simulink model "HIL_Testing_SW_amantest"  (Simulink 7.5)
settings: Solver=ode1  StartTime=0.0  StopTime=Inf  FixedStep=0.001  RelTol=1e-3
PostLoadFcn:
  | , if any(exist('dsrtsu_mdlpostloadfcn', 'file') == [2, 3, 6]), try dsrtsu_mdlpostloadfcn('Execute', bdroot); catch fprintf('Error in PostLoadFcn (dsrtsu_mdlpostloadfcn) for model "%s":\n %s\n', bdroot, lasterr); end, end,
undefined symbols (not defined in the file): CeBSER_Cnt_NumTempAxisPts, ChargeCord, ChargeCord_Control, ChargeToSOCCurr, ChrgCurrLim, CrntSens1Fine, CS_SOCSetPt, CyclerMaxChrgPwr, CyclerMaxDschrgPwr, deltaAhr, Drive_1, Drive_10, Drive_11, Drive_12, Drive_13, Drive_14, Drive_15, Drive_16, Drive_17, Drive_18, Drive_19, Drive_2, Drive_20, Drive_21, Drive_22, Drive_23, Drive_24, Drive_25, Drive_26, Drive_27, Drive_28, Drive_29, Drive_3, Drive_30, Drive_31, Drive_32, Drive_33, Drive_34, Drive_35, Drive_36, Drive_37, Drive_38, Drive_39, Drive_4, Drive_40, Drive_41, Drive_42, Drive_43, Drive_44, Drive_45, Drive_46, Drive_47, Drive_48, Drive_49, Drive_5, Drive_50, Drive_51, Drive_6, Drive_7, Drive_8 ... (+50)
libraries: simulink x129, rtican x50, rti2211sailib x5, rti2211serlib x5, rti2202miolib x3
(part 8 of 23)

== system HIL_Testing_SW_amantest/RX/Read BAS3/Read PTEX ==
  PPEI_High_Vlt_Battery_Vlt_Status1 : rtican/RTICAN Receive (RX)   SystemSampleTime=-1  Reserved1=[]  Reserved2=[]  Reserved3=[]  Reserved4=[]  SfcnMessage=[]  Msg_Struct=[]  BoardTypeNo=[]  BoardNo=[]  ChannelNo=[]  Parameters=[]  DialogFcn=[]  UnitName=[]  Revision=[]  UnitValues=[]  DSProperties=struct('RTI',struct('Version',uint32(5),'BlockType',struct('isSLSource',uint8(1),'isSLSink',uint8(1),'isHWSource',uint8(0),'isHWSink',uint8(0),'isSetup',uint8(0),'isInline',uint8(1),'isNonInline',uint8(0),'isInterrupt',uint8(0),'isChannelwise',uint8(0)),'IOBoardType','RTICAN','UnitType','MESSAGE','Identifier','RX','DialogType','MSVC','BlockSet','RTICAN','SlaveProcessor','CAN'))  RTIBlockInterface=struct('OutputPortsWidth',int32([1 1 1 1 1 1 1 1]),'OutputPortsActive',[1 1 1 1 1 1 1 1],'OutputPortsName',{{'HVBatVltLwLmtCrnk','HVBatVltLwLmtCrnkV','HVBatVltLwLmt','HVBatVltLwLmtV','HVBatVltUpLmt','HVBatVltUpLmtV','HVBatPackPrcdVltg','HVBatPackPrcdVltgV'}},'OutputPortsDataType',{{'SS_DOUBLE','SS_DOUBLE','SS_DOUBLE','SS_DOUBLE','SS_DOUBLE','SS_DOUBLE','SS_DOUBLE','SS_DOUBLE'}},'OutputPortsLabel',{{'HVBatVltLwLmtCrnk','HVBatVltLwLmtCrnkV','HVBatVltLwLmt','HVBatVltLwLmtV','HVBatVltUpLmt','HVBatVltUpLmtV','HVBatPackPrcdVltg','HVBatPackPrcdVltgV'}},'OutputPortsLabelMode','ON','InputPortsWidth',int32(0),'InputPortsActive',0,'DialogFcn','rtican_message_interface_gui','BlockDisplay',{{'','center'}},'IconTransparency','on','ParameterTunableNames',{{}},'InitLevel',3,'BlockName',struct('Token',{{'PPEI_High_Vlt_Battery_Vlt_Status'}}),'SampleTime',{{-1}},'TriggerPort',{{'none'}},'EnablePort',{{'none'}})  RTIBlockParameters=struct('BoardTypeNo',{{4302,'OFF',[]}},'BoardNo',{{1,'ON',[1 16]}},'ChannelNo',{{2,'ON',[1 4]}},'Parameters',{{struct('DataFileSupport',struct('DataFileSelectedMaster',1,'DataFileSelectedLocal',1,'DataFileName',['c:\data\databases\6.4.1\globala - pe.dbc|'],'DataFileDate',['24-Apr-2014 15:33:48'],'SelectedFile',['..\databases\8.4.5 (140425)\globala - pe.dbc'],'InterfaceFcn','rtican_dbc_file_parser'),'Options',struct('StatusSelected',0,'TimeSelected',0,'DeltaTimeSelected',0,'BytePortSelected',0,'MessageLengthSelected',0,'TriggerPort',struct('Selected',0,'TriggerType',0),'UserCoding',struct('Selected',0,'InterfaceFile','UserDecodingFile','FcnName','UserDecodeFcn','InportSelected',0,'InportWidth',1,'OutportSelected',0,'OutportWidth',1),'EnablePortSelected',0,'SignalOnPortnameSelected',1,'UseRXService',0),'Message',struct('MsgOnBlocknameSelected',1,'MsgName','PPEI_High_Vlt_Battery_Vlt_Status','MsgIdFormat',0,'MsgId',983,'MsgLength',8,'NumSignals',8,'SampleTime',-1,'Signal',struct('SgnName',{'HVBatVltLwLmtCrnk','HVBatVltLwLmtCrnkV','HVBatVltLwLmt','HVBatVltLwLmtV','HVBatVltUpLmt','HVBatVltUpLmtV','HVBatPackPrcdVltg','HVBatPackPrcdVltgV'},'SgnStartBit',{0,10,16,26,32,42,48,58},'SgnLength',{10,1,10,1,10,1,10,1},'ByteLayout',{2,2,2,2,2,2,2,2},'Factor',{0.52,1,0.52,1,0.52,1,0.52,1},'Offset',{0,0,0,0,0,0,0,0},'SgnComment',{'','','','','','','',''},'SgnUnit',{'V','','V','','V','','V',''},'Min',{0,0,0,0,0,0,0,0},'Max',{531.96,1,531.96,1,531.96,1,531.96,1},'SgnType',{0,0,0,0,0,0,0,0},'SLDataType',{'SS_DOUBLE','SS_DOUBLE','SS_DOUBLE','SS_DOUBLE','SS_DOUBLE','SS_DOUBLE','SS_DOUBLE','SS_DOUBLE'},'DataType',{0,0,0,0,0,0,0,0},'ModeValue',{-1,-1,-1,-1,-1,-1,-1,-1}),'MsgIdNumFormat',0,'MsgComment',{{''}}),'Version',1.2,'general',struct('isFromLib',0)),'OFF',[]}},'GroupId',{{struct('Group',{{'RTICAN'}},'No',5,'Behavior',{{'NAMECHANGE'}},'BlockType',{{'SINK'}},'NameChangeFlag',0),'OFF',[]}},'SFcnRTICANMessage',{{struct('MsgType','RX','SFcnPortType','Scalar','MsgName','PPEI_High_Vlt_Battery_Vlt_Status','MsgIdFormat','STD','MsgId',983,'MsgLength',8,'NumSignals',8,'SampleTime',-1,'Signal',struct('SgnName',{'HVBatVltLwLmtCrnk','HVBatVltLwLmtCrnkV','HVBatVltLwLmt','HVBatVltLwLmtV','HVBatVltUpLmt','HVBatVltUpLmtV','HVBatPackPrcdVltg','HVBatPackPrcdVltgV'},'SgnStartBit',{0,10,16,26,32,42,48,58},'SgnLength',{10,1,10,1,10,1,10,1},'ByteLayout',{['motorola back.'],['motorola back.'],['motorola back.'],['motorola back.'],['motorola back.'],['motorola back.'],['motorola back.'],['motorola back.']},'Factor',{0.52,1,0.52,1,0.52,1,0.52,1},'Offset',{0,0,0,0,0,0,0,0},'SgnType',{'standard','standard','standard','standard','standard','standard','standard','standard'},'SLDataType',{'SS_DOUBLE','SS_DOUBLE','SS_DOUBLE','SS_DOUBLE','SS_DOUBLE','SS_DOUBLE','SS_DOUBLE','SS_DOUBLE'},'DataType',{['unsigned int'],['unsigned int'],['unsigned int'],['unsigned int'],['unsigned int'],['unsigned int'],['unsigned int'],['unsigned int']},'ModeValue',{-1,-1,-1,-1,-1,-1,-1,-1}),'StatusSelected','no','TimeSelected','no','DeltaTimeSelected','no','BytePortSelected','no','MessageLengthSelected','no','TriggerPort',struct('Selected','no','TriggerType',0),'UserCoding',struct('Selected','no','InterfaceFile','UserDecodingFile','FcnName','UserDecodeFcn','InportSelected','no','InportWidth',1,'OutportSelected','no','OutportWidth',1),'EnablePortSelected','no','UseRXService','no','BoardType','DS4302','BoardNo',1,'ControllerNo',2),'OFF',[]}},'TLCFileName',{{'rtican_rx_message','OFF',[]}})  RTISFcnParameters=struct('SFcnRTICANMessage','struct','TLCFileName','char')  RTIBlockParaDefault=struct('BoardTypeNo',4302,'BoardNo',1,'ChannelNo',1,'Parameters',struct('DataFileSupport',struct('DataFileSelectedMaster',0,'DataFileSelectedLocal',0,'DataFileName','','DataFileDate','','SelectedFile',['<no file selected>']),'Options',struct('StatusSelected',1,'TimeSelected',1,'DeltaTimeSelected',1,'BytePortSelected',0,'MessageLengthSelected',0,'TriggerPort',struct('Selected',0,'TriggerType','rising'),'UserCoding',struct('Selected',0,'InterfaceFile','UserDecodingFile','FcnName','UserDecodeFcn','InportSelected',0,'InportWidth',1,'OutportSelected',0,'OutportWidth',1),'EnablePortSelected',0,'SignalOnPortnameSelected',1,'UseRXService',0),'Message',struct('MsgOnBlocknameSelected',0,'MsgName',['RX Message'],'MsgIdFormat',0,'MsgId',100,'MsgLength',8,'NumSignals',1,'SampleTime',-1,'Signal',struct('SgnName',['RX signal'],'SgnStartBit',0,'SgnLength',8,'SgnType',0,'ModeValue',-1,'DataType',0,'SLDataType','SS_DOUBLE','ByteLayout',0,'Factor',1,'Offset',0,'Min',0,'Max',255,'SgnComment',{{}},'SgnUnit',''),'MsgIdNumFormat',0,'MsgComment',{{''}}),'Version',1.2,'general',struct('isFromLib',1)),'GroupId',struct('Group',{{'RTICAN'}},'No',1,'Behavior',{{'NAMECHANGE'}},'BlockType',{{'SINK'}},'NameChangeFlag',0),'SFcnRTICANMessage',struct('MsgType','RX','MsgName',['RX Message'],'MsgIdFormat','STD','MsgId',100,'MsgLength',8,'NumSignals',1,'SampleTime',-1,'Signal',struct('SgnName',['RX signal'],'SgnStartBit',0,'SgnLength',8,'SgnType','standard','ModeValue',-1,'DataType',['unsigned int'],'ByteLayout',['little endian'],'SLDataType','SS_DOUBLE','Factor',1,'Offset',0),'StatusSelected','yes','TimeSelected','yes','DeltaTimeSelected','yes','BytePortSelected','no','MessageLengthSelected','no','EnablePortSelected','no','UserCoding',struct('Selected','no','InterfaceFile','UserDecodingFile','FcnName','UserDecodeFcn','InportSelected','no','InportWidth',1,'OutportSelected','no','OutportWidth',1),'TriggerPort',struct('Selected','no','TriggerType','rising'),'UseRXService','no','BoardType','DS4302','BoardNo',1,'ControllerNo',1,'SFcnPortType','Scalar'),'TLCFileName','rtican_rx_message')
      settings: AttributesFormatString=Group Id: RTICAN5\n
  PPEI_High_Volt_Batt_Current_Stat1 : rtican/RTICAN Receive (RX)   SystemSampleTime=-1  Reserved1=[]  Reserved2=[]  Reserved3=[]  Reserved4=[]  SfcnMessage=[]  Msg_Struct=[]  BoardTypeNo=[]  BoardNo=[]  ChannelNo=[]  Parameters=[]  DialogFcn=[]  UnitName=[]  Revision=[]  UnitValues=[]  DSProperties=struct('RTI',struct('Version',uint32(5),'BlockType',struct('isSLSource',uint8(1),'isSLSink',uint8(1),'isHWSource',uint8(0),'isHWSink',uint8(0),'isSetup',uint8(0),'isInline',uint8(1),'isNonInline',uint8(0),'isInterrupt',uint8(0),'isChannelwise',uint8(0)),'IOBoardType','RTICAN','UnitType','MESSAGE','Identifier','RX','DialogType','MSVC','BlockSet','RTICAN','SlaveProcessor','CAN'))  RTIBlockInterface=struct('OutputPortsWidth',int32([1 1 1 1 1 1]),'OutputPortsActive',[1 1 1 1 1 1],'OutputPortsName',{{'HVBatStOfChrgMin','HVBatCrntLwLmt','HVBatCrntLwLmtV','HVBatCrntUpLmt','HVBatCrntUpLmtV','HVBatSOCTrgtHiRes'}},'OutputPortsDataType',{{'SS_DOUBLE','SS_DOUBLE','SS_DOUBLE','SS_DOUBLE','SS_DOUBLE','SS_DOUBLE'}},'OutputPortsLabel',{{'HVBatStOfChrgMin','HVBatCrntLwLmt','HVBatCrntLwLmtV','HVBatCrntUpLmt','HVBatCrntUpLmtV','HVBatSOCTrgtHiRes'}},'OutputPortsLabelMode','ON','InputPortsWidth',int32(0),'InputPortsActive',0,'DialogFcn','rtican_message_interface_gui','BlockDisplay',{{'','center'}},'IconTransparency','on','ParameterTunableNames',{{}},'InitLevel',3,'BlockName',struct('Token',{{'PPEI_High_Volt_Batt_Current_Stat'}}),'SampleTime',{{-1}},'TriggerPort',{{'none'}},'EnablePort',{{'none'}})  RTIBlockParameters=struct('BoardTypeNo',{{4302,'OFF',[]}},'BoardNo',{{1,'ON',[1 16]}},'ChannelNo',{{2,'ON',[1 4]}},'Parameters',{{struct('DataFileSupport',struct('DataFileSelectedMaster',1,'DataFileSelectedLocal',1,'DataFileName',['c:\data\databases\6.4.1\globala - pe.dbc|'],'DataFileDate',['24-Apr-2014 15:33:48'],'SelectedFile',['..\databases\8.4.5 (140425)\globala - pe.dbc'],'InterfaceFcn','rtican_dbc_file_parser'),'Options',struct('StatusSelected',0,'TimeSelected',0,'DeltaTimeSelected',0,'BytePortSelected',0,'MessageLengthSelected',0,'TriggerPort',struct('Selected',0,'TriggerType',0),'UserCoding',struct('Selected',0,'InterfaceFile','UserDecodingFile','FcnName','UserDecodeFcn','InportSelected',0,'InportWidth',1,'OutportSelected',0,'OutportWidth',1),'EnablePortSelected',0,'SignalOnPortnameSelected',1,'UseRXService',0),'Message',struct('MsgOnBlocknameSelected',1,'MsgName','PPEI_High_Volt_Batt_Current_Stat','MsgIdFormat',0,'MsgId',981,'MsgLength',8,'NumSignals',6,'SampleTime',-1,'Signal',struct('SgnName',{'HVBatStOfChrgMin','HVBatCrntLwLmt','HVBatCrntLwLmtV','HVBatCrntUpLmt','HVBatCrntUpLmtV','HVBatSOCTrgtHiRes'},'SgnStartBit',{0,16,27,32,43,48},'SgnLength',{8,11,1,11,1,16},'ByteLayout',{2,2,2,2,2,2},'Factor',{0.392157,0.3,1,0.3,1,0.001526},'Offset',{0,0,0,0,0,0},'SgnComment',{'','','','','',''},'SgnUnit',{'','A','','A','','%'},'Min',{0,0,0,0,0,0},'Max',{100.000035,614.1,1,614.1,1,100},'SgnType',{0,0,0,0,0,0},'SLDataType',{'SS_DOUBLE','SS_DOUBLE','SS_DOUBLE','SS_DOUBLE','SS_DOUBLE','SS_DOUBLE'},'DataType',{0,0,0,0,0,0},'ModeValue',{-1,-1,-1,-1,-1,-1}),'MsgIdNumFormat',0,'MsgComment',{{''}}),'Version',1.2,'general',struct('isFromLib',0)),'OFF',[]}},'GroupId',{{struct('Group',{{'RTICAN'}},'No',5,'Behavior',{{'NAMECHANGE'}},'BlockType',{{'SINK'}},'NameChangeFlag',0),'OFF',[]}},'SFcnRTICANMessage',{{struct('MsgType','RX','SFcnPortType','Scalar','MsgName','PPEI_High_Volt_Batt_Current_Stat','MsgIdFormat','STD','MsgId',981,'MsgLength',8,'NumSignals',6,'SampleTime',-1,'Signal',struct('SgnName',{'HVBatStOfChrgMin','HVBatCrntLwLmt','HVBatCrntLwLmtV','HVBatCrntUpLmt','HVBatCrntUpLmtV','HVBatSOCTrgtHiRes'},'SgnStartBit',{0,16,27,32,43,48},'SgnLength',{8,11,1,11,1,16},'ByteLayout',{['motorola back.'],['motorola back.'],['motorola back.'],['motorola back.'],['motorola back.'],['motorola back.']},'Factor',{0.392157,0.3,1,0.3,1,0.001526},'Offset',{0,0,0,0,0,0},'SgnType',{'standard','standard','standard','standard','standard','standard'},'SLDataType',{'SS_DOUBLE','SS_DOUBLE','SS_DOUBLE','SS_DOUBLE','SS_DOUBLE','SS_DOUBLE'},'DataType',{['unsigned int'],['unsigned int'],['unsigned int'],['unsigned int'],['unsigned int'],['unsigned int']},'ModeValue',{-1,-1,-1,-1,-1,-1}),'StatusSelected','no','TimeSelected','no','DeltaTimeSelected','no','BytePortSelected','no','MessageLengthSelected','no','TriggerPort',struct('Selected','no','TriggerType',0),'UserCoding',struct('Selected','no','InterfaceFile','UserDecodingFile','FcnName','UserDecodeFcn','InportSelected','no','InportWidth',1,'OutportSelected','no','OutportWidth',1),'EnablePortSelected','no','UseRXService','no','BoardType','DS4302','BoardNo',1,'ControllerNo',2),'OFF',[]}},'TLCFileName',{{'rtican_rx_message','OFF',[]}})  RTISFcnParameters=struct('SFcnRTICANMessage','struct','TLCFileName','char')  RTIBlockParaDefault=struct('BoardTypeNo',4302,'BoardNo',1,'ChannelNo',1,'Parameters',struct('DataFileSupport',struct('DataFileSelectedMaster',0,'DataFileSelectedLocal',0,'DataFileName','','DataFileDate','','SelectedFile',['<no file selected>']),'Options',struct('StatusSelected',1,'TimeSelected',1,'DeltaTimeSelected',1,'BytePortSelected',0,'MessageLengthSelected',0,'TriggerPort',struct('Selected',0,'TriggerType','rising'),'UserCoding',struct('Selected',0,'InterfaceFile','UserDecodingFile','FcnName','UserDecodeFcn','InportSelected',0,'InportWidth',1,'OutportSelected',0,'OutportWidth',1),'EnablePortSelected',0,'SignalOnPortnameSelected',1,'UseRXService',0),'Message',struct('MsgOnBlocknameSelected',0,'MsgName',['RX Message'],'MsgIdFormat',0,'MsgId',100,'MsgLength',8,'NumSignals',1,'SampleTime',-1,'Signal',struct('SgnName',['RX signal'],'SgnStartBit',0,'SgnLength',8,'SgnType',0,'ModeValue',-1,'DataType',0,'SLDataType','SS_DOUBLE','ByteLayout',0,'Factor',1,'Offset',0,'Min',0,'Max',255,'SgnComment',{{}},'SgnUnit',''),'MsgIdNumFormat',0,'MsgComment',{{''}}),'Version',1.2,'general',struct('isFromLib',1)),'GroupId',struct('Group',{{'RTICAN'}},'No',1,'Behavior',{{'NAMECHANGE'}},'BlockType',{{'SINK'}},'NameChangeFlag',0),'SFcnRTICANMessage',struct('MsgType','RX','MsgName',['RX Message'],'MsgIdFormat','STD','MsgId',100,'MsgLength',8,'NumSignals',1,'SampleTime',-1,'Signal',struct('SgnName',['RX signal'],'SgnStartBit',0,'SgnLength',8,'SgnType','standard','ModeValue',-1,'DataType',['unsigned int'],'ByteLayout',['little endian'],'SLDataType','SS_DOUBLE','Factor',1,'Offset',0),'StatusSelected','yes','TimeSelected','yes','DeltaTimeSelected','yes','BytePortSelected','no','MessageLengthSelected','no','EnablePortSelected','no','UserCoding',struct('Selected','no','InterfaceFile','UserDecodingFile','FcnName','UserDecodeFcn','InportSelected','no','InportWidth',1,'OutportSelected','no','OutportWidth',1),'TriggerPort',struct('Selected','no','TriggerType','rising'),'UseRXService','no','BoardType','DS4302','BoardNo',1,'ControllerNo',1,'SFcnPortType','Scalar'),'TLCFileName','rtican_rx_message')
      settings: AttributesFormatString=Group Id: RTICAN5\n
  PPEI_High_Volt_Batt_Dchrg_Pwrs1 : rtican/RTICAN Receive (RX)   SystemSampleTime=-1  Reserved1=[]  Reserved2=[]  Reserved3=[]  Reserved4=[]  SfcnMessage=[]  Msg_Struct=[]  BoardTypeNo=[]  BoardNo=[]  ChannelNo=[]  Parameters=[]  DialogFcn=[]  UnitName=[]  Revision=[]  UnitValues=[]  DSProperties=struct('RTI',struct('Version',uint32(5),'BlockType',struct('isSLSource',uint8(1),'isSLSink',uint8(1),'isHWSource',uint8(0),'isHWSink',uint8(0),'isSetup',uint8(0),'isInline',uint8(1),'isNonInline',uint8(0),'isInterrupt',uint8(0),'isChannelwise',uint8(0)),'IOBoardType','RTICAN','UnitType','MESSAGE','Identifier','RX','DialogType','MSVC','BlockSet','RTICAN','SlaveProcessor','CAN'))  RTIBlockInterface=struct('OutputPortsWidth',int32([1 1 1 1 1]),'OutputPortsActive',[1 1 1 1 1],'OutputPortsName',{{'HVBDP_ShrtTrmDischrgPwr','HVBDP_CrnkDischrgPwrV','HVBDP_Res','HVBDP_LngTrmDischrgPwr','HVBDP_CrnkDischrgPwr'}},'OutputPortsDataType',{{'SS_DOUBLE','SS_DOUBLE','SS_DOUBLE','SS_DOUBLE','SS_DOUBLE'}},'OutputPortsLabel',{{'HVBDP_ShrtTrmDischrgPwr','HVBDP_CrnkDischrgPwrV','HVBDP_Res','HVBDP_LngTrmDischrgPwr','HVBDP_CrnkDischrgPwr'}},'OutputPortsLabelMode','ON','InputPortsWidth',int32(0),'InputPortsActive',0,'DialogFcn','rtican_message_interface_gui','BlockDisplay',{{'','center'}},'IconTransparency','on','ParameterTunableNames',{{}},'InitLevel',3,'BlockName',struct('Token',{{'PPEI_High_Volt_Batt_Dchrg_Pwrs'}}),'SampleTime',{{-1}},'TriggerPort',{{'none'}},'EnablePort',{{'none'}})  RTIBlockParameters=struct('BoardTypeNo',{{4302,'OFF',[]}},'BoardNo',{{1,'ON',[1 16]}},'ChannelNo',{{2,'ON',[1 4]}},'Parameters',{{struct('DataFileSupport',struct('DataFileSelectedMaster',1,'DataFileSelectedLocal',1,'DataFileName',['c:\data\databases\6.4.1\globala - pe.dbc|'],'DataFileDate',['24-Apr-2014 15:33:48'],'SelectedFile',['..\databases\8.4.5 (140425)\globala - pe.dbc'],'InterfaceFcn','rtican_dbc_file_parser'),'Options',struct('StatusSelected',0,'TimeSelected',0,'DeltaTimeSelected',0,'BytePortSelected',0,'MessageLengthSelected',0,'TriggerPort',struct('Selected',0,'TriggerType',0),'UserCoding',struct('Selected',0,'InterfaceFile','UserDecodingFile','FcnName','UserDecodeFcn','InportSelected',0,'InportWidth',1,'OutportSelected',0,'OutportWidth',1),'EnablePortSelected',0,'SignalOnPortnameSelected',1,'UseRXService',0),'Message',struct('MsgOnBlocknameSelected',1,'MsgName','PPEI_High_Volt_Batt_Dchrg_Pwrs','MsgIdFormat',0,'MsgId',987,'MsgLength',6,'NumSignals',5,'SampleTime',-1,'Signal',struct('SgnName',{'HVBDP_ShrtTrmDischrgPwr','HVBDP_CrnkDischrgPwrV','HVBDP_Res','HVBDP_LngTrmDischrgPwr','HVBDP_CrnkDischrgPwr'},'SgnStartBit',{13,24,25,26,37},'SgnLength',{11,1,1,11,11},'ByteLayout',{2,2,2,2,2},'Factor',{0.1,1,1,0.1,0.1},'Offset',{0,0,0,0,0},'SgnComment',{'','','','',''},'SgnUnit',{'kW','','','kW','kW'},'Min',{0,0,0,0,0},'Max',{204.7,1,1,204.7,204.7},'SgnType',{0,0,0,0,0},'SLDataType',{'SS_DOUBLE','SS_DOUBLE','SS_DOUBLE','SS_DOUBLE','SS_DOUBLE'},'DataType',{0,0,0,0,0},'ModeValue',{-1,-1,-1,-1,-1}),'MsgIdNumFormat',0,'MsgComment',{{''}}),'Version',1.2,'general',struct('isFromLib',0)),'OFF',[]}},'GroupId',{{struct('Group',{{'RTICAN'}},'No',5,'Behavior',{{'NAMECHANGE'}},'BlockType',{{'SINK'}},'NameChangeFlag',0),'OFF',[]}},'SFcnRTICANMessage',{{struct('MsgType','RX','SFcnPortType','Scalar','MsgName','PPEI_High_Volt_Batt_Dchrg_Pwrs','MsgIdFormat','STD','MsgId',987,'MsgLength',6,'NumSignals',5,'SampleTime',-1,'Signal',struct('SgnName',{'HVBDP_ShrtTrmDischrgPwr','HVBDP_CrnkDischrgPwrV','HVBDP_Res','HVBDP_LngTrmDischrgPwr','HVBDP_CrnkDischrgPwr'},'SgnStartBit',{13,24,25,26,37},'SgnLength',{11,1,1,11,11},'ByteLayout',{['motorola back.'],['motorola back.'],['motorola back.'],['motorola back.'],['motorola back.']},'Factor',{0.1,1,1,0.1,0.1},'Offset',{0,0,0,0,0},'SgnType',{'standard','standard','standard','standard','standard'},'SLDataType',{'SS_DOUBLE','SS_DOUBLE','SS_DOUBLE','SS_DOUBLE','SS_DOUBLE'},'DataType',{['unsigned int'],['unsigned int'],['unsigned int'],['unsigned int'],['unsigned int']},'ModeValue',{-1,-1,-1,-1,-1}),'StatusSelected','no','TimeSelected','no','DeltaTimeSelected','no','BytePortSelected','no','MessageLengthSelected','no','TriggerPort',struct('Selected','no','TriggerType',0),'UserCoding',struct('Selected','no','InterfaceFile','UserDecodingFile','FcnName','UserDecodeFcn','InportSelected','no','InportWidth',1,'OutportSelected','no','OutportWidth',1),'EnablePortSelected','no','UseRXService','no','BoardType','DS4302','BoardNo',1,'ControllerNo',2),'OFF',[]}},'TLCFileName',{{'rtican_rx_message','OFF',[]}})  RTISFcnParameters=struct('SFcnRTICANMessage','struct','TLCFileName','char')  RTIBlockParaDefault=struct('BoardTypeNo',4302,'BoardNo',1,'ChannelNo',1,'Parameters',struct('DataFileSupport',struct('DataFileSelectedMaster',0,'DataFileSelectedLocal',0,'DataFileName','','DataFileDate','','SelectedFile',['<no file selected>']),'Options',struct('StatusSelected',1,'TimeSelected',1,'DeltaTimeSelected',1,'BytePortSelected',0,'MessageLengthSelected',0,'TriggerPort',struct('Selected',0,'TriggerType','rising'),'UserCoding',struct('Selected',0,'InterfaceFile','UserDecodingFile','FcnName','UserDecodeFcn','InportSelected',0,'InportWidth',1,'OutportSelected',0,'OutportWidth',1),'EnablePortSelected',0,'SignalOnPortnameSelected',1,'UseRXService',0),'Message',struct('MsgOnBlocknameSelected',0,'MsgName',['RX Message'],'MsgIdFormat',0,'MsgId',100,'MsgLength',8,'NumSignals',1,'SampleTime',-1,'Signal',struct('SgnName',['RX signal'],'SgnStartBit',0,'SgnLength',8,'SgnType',0,'ModeValue',-1,'DataType',0,'SLDataType','SS_DOUBLE','ByteLayout',0,'Factor',1,'Offset',0,'Min',0,'Max',255,'SgnComment',{{}},'SgnUnit',''),'MsgIdNumFormat',0,'MsgComment',{{''}}),'Version',1.2,'general',struct('isFromLib',1)),'GroupId',struct('Group',{{'RTICAN'}},'No',1,'Behavior',{{'NAMECHANGE'}},'BlockType',{{'SINK'}},'NameChangeFlag',0),'SFcnRTICANMessage',struct('MsgType','RX','MsgName',['RX Message'],'MsgIdFormat','STD','MsgId',100,'MsgLength',8,'NumSignals',1,'SampleTime',-1,'Signal',struct('SgnName',['RX signal'],'SgnStartBit',0,'SgnLength',8,'SgnType','standard','ModeValue',-1,'DataType',['unsigned int'],'ByteLayout',['little endian'],'SLDataType','SS_DOUBLE','Factor',1,'Offset',0),'StatusSelected','yes','TimeSelected','yes','DeltaTimeSelected','yes','BytePortSelected','no','MessageLengthSelected','no','EnablePortSelected','no','UserCoding',struct('Selected','no','InterfaceFile','UserDecodingFile','FcnName','UserDecodeFcn','InportSelected','no','InportWidth',1,'OutportSelected','no','OutportWidth',1),'TriggerPort',struct('Selected','no','TriggerType','rising'),'UseRXService','no','BoardType','DS4302','BoardNo',1,'ControllerNo',1,'SFcnPortType','Scalar'),'TLCFileName','rtican_rx_message')
      settings: AttributesFormatString=Group Id: RTICAN5\n
  PPEI_High_Voltage_Batt_Chrg_Pwrs1 : rtican/RTICAN Receive (RX)   SystemSampleTime=-1  Reserved1=[]  Reserved2=[]  Reserved3=[]  Reserved4=[]  SfcnMessage=[]  Msg_Struct=[]  BoardTypeNo=[]  BoardNo=[]  ChannelNo=[]  Parameters=[]  DialogFcn=[]  UnitName=[]  Revision=[]  UnitValues=[]  DSProperties=struct('RTI',struct('Version',uint32(5),'BlockType',struct('isSLSource',uint8(1),'isSLSink',uint8(1),'isHWSource',uint8(0),'isHWSink',uint8(0),'isSetup',uint8(0),'isInline',uint8(1),'isNonInline',uint8(0),'isInterrupt',uint8(0),'isChannelwise',uint8(0)),'IOBoardType','RTICAN','UnitType','MESSAGE','Identifier','RX','DialogType','MSVC','BlockSet','RTICAN','SlaveProcessor','CAN'))  RTIBlockInterface=struct('OutputPortsWidth',int32([1 1 1 1 1 1 1 1]),'OutputPortsActive',[1 1 1 1 1 1 1 1],'OutputPortsName',{{'HVBatSOCHiRes','HVBatOutOfEnrgyStat','HVBatSOCHiResV','HVBCP_ShrtTrmChrgPwr','HVBCP_CrnkChrgPwrV','HVBCP_Res','HVBCP_LngTrmChrgPwr','HVBCP_CrnkChrgPwr'}},'OutputPortsDataType',{{'SS_DOUBLE','SS_DOUBLE','SS_DOUBLE','SS_DOUBLE','SS_DOUBLE','SS_DOUBLE','SS_DOUBLE','SS_DOUBLE'}},'OutputPortsLabel',{{'HVBatSOCHiRes','HVBatOutOfEnrgyStat','HVBatSOCHiResV','HVBCP_ShrtTrmChrgPwr','HVBCP_CrnkChrgPwrV','HVBCP_Res','HVBCP_LngTrmChrgPwr','HVBCP_CrnkChrgPwr'}},'OutputPortsLabelMode','ON','InputPortsWidth',int32(0),'InputPortsActive',0,'DialogFcn','rtican_message_interface_gui','BlockDisplay',{{'','center'}},'IconTransparency','on','ParameterTunableNames',{{}},'InitLevel',3,'BlockName',struct('Token',{{'PPEI_High_Voltage_Batt_Chrg_Pwrs'}}),'SampleTime',{{-1}},'TriggerPort',{{'none'}},'EnablePort',{{'none'}})  RTIBlockParameters=struct('BoardTypeNo',{{4302,'OFF',[]}},'BoardNo',{{1,'ON',[1 16]}},'ChannelNo',{{2,'ON',[1 4]}},'Parameters',{{struct('DataFileSupport',struct('DataFileSelectedMaster',1,'DataFileSelectedLocal',1,'DataFileName',['c:\data\databases\6.4.1\globala - pe.dbc|'],'DataFileDate',['24-Apr-2014 15:33:48'],'SelectedFile',['..\databases\8.4.5 (140425)\globala - pe.dbc'],'InterfaceFcn','rtican_dbc_file_parser'),'Options',struct('StatusSelected',0,'TimeSelected',0,'DeltaTimeSelected',0,'BytePortSelected',0,'MessageLengthSelected',0,'TriggerPort',struct('Selected',0,'TriggerType',0),'UserCoding',struct('Selected',0,'InterfaceFile','UserDecodingFile','FcnName','UserDecodeFcn','InportSelected',0,'InportWidth',1,'OutportSelected',0,'OutportWidth',1),'EnablePortSelected',0,'SignalOnPortnameSelected',1,'UseRXService',0),'Message',struct('MsgOnBlocknameSelected',1,'MsgName','PPEI_High_Voltage_Batt_Chrg_Pwrs','MsgIdFormat',0,'MsgId',986,'MsgLength',8,'NumSignals',8,'SampleTime',-1,'Signal',struct('SgnName',{'HVBatSOCHiRes','HVBatOutOfEnrgyStat','HVBatSOCHiResV','HVBCP_ShrtTrmChrgPwr','HVBCP_CrnkChrgPwrV','HVBCP_Res','HVBCP_LngTrmChrgPwr','HVBCP_CrnkChrgPwr'},'SgnStartBit',{0,25,28,29,40,41,42,53},'SgnLength',{16,3,1,11,1,1,11,11},'ByteLayout',{2,2,2,2,2,2,2,2},'Factor',{0.00152593,1,1,0.1,1,1,0.1,0.1},'Offset',{0,0,0,0,0,0,0,0},'SgnComment',{'','','','','','','',''},'SgnUnit',{'%','','','kW','','','kW','kW'},'Min',{0,0,0,0,0,0,0,0},'Max',{100.00182255,7,1,204.7,1,1,204.7,204.7},'SgnType',{0,0,0,0,0,0,0,0},'SLDataType',{'SS_DOUBLE','SS_DOUBLE','SS_DOUBLE','SS_DOUBLE','SS_DOUBLE','SS_DOUBLE','SS_DOUBLE','SS_DOUBLE'},'DataType',{0,0,0,0,0,0,0,0},'ModeValue',{-1,-1,-1,-1,-1,-1,-1,-1}),'MsgIdNumFormat',0,'MsgComment',{{''}}),'Version',1.2,'general',struct('isFromLib',0)),'OFF',[]}},'GroupId',{{struct('Group',{{'RTICAN'}},'No',5,'Behavior',{{'NAMECHANGE'}},'BlockType',{{'SINK'}},'NameChangeFlag',0),'OFF',[]}},'SFcnRTICANMessage',{{struct('MsgType','RX','SFcnPortType','Scalar','MsgName','PPEI_High_Voltage_Batt_Chrg_Pwrs','MsgIdFormat','STD','MsgId',986,'MsgLength',8,'NumSignals',8,'SampleTime',-1,'Signal',struct('SgnName',{'HVBatSOCHiRes','HVBatOutOfEnrgyStat','HVBatSOCHiResV','HVBCP_ShrtTrmChrgPwr','HVBCP_CrnkChrgPwrV','HVBCP_Res','HVBCP_LngTrmChrgPwr','HVBCP_CrnkChrgPwr'},'SgnStartBit',{0,25,28,29,40,41,42,53},'SgnLength',{16,3,1,11,1,1,11,11},'ByteLayout',{['motorola back.'],['motorola back.'],['motorola back.'],['motorola back.'],['motorola back.'],['motorola back.'],['motorola back.'],['motorola back.']},'Factor',{0.00152593,1,1,0.1,1,1,0.1,0.1},'Offset',{0,0,0,0,0,0,0,0},'SgnType',{'standard','standard','standard','standard','standard','standard','standard','standard'},'SLDataType',{'SS_DOUBLE','SS_DOUBLE','SS_DOUBLE','SS_DOUBLE','SS_DOUBLE','SS_DOUBLE','SS_DOUBLE','SS_DOUBLE'},'DataType',{['unsigned int'],['unsigned int'],['unsigned int'],['unsigned int'],['unsigned int'],['unsigned int'],['unsigned int'],['unsigned int']},'ModeValue',{-1,-1,-1,-1,-1,-1,-1,-1}),'StatusSelected','no','TimeSelected','no','DeltaTimeSelected','no','BytePortSelected','no','MessageLengthSelected','no','TriggerPort',struct('Selected','no','TriggerType',0),'UserCoding',struct('Selected','no','InterfaceFile','UserDecodingFile','FcnName','UserDecodeFcn','InportSelected','no','InportWidth',1,'OutportSelected','no','OutportWidth',1),'EnablePortSelected','no','UseRXService','no','BoardType','DS4302','BoardNo',1,'ControllerNo',2),'OFF',[]}},'TLCFileName',{{'rtican_rx_message','OFF',[]}})  RTISFcnParameters=struct('SFcnRTICANMessage','struct','TLCFileName','char')  RTIBlockParaDefault=struct('BoardTypeNo',4302,'BoardNo',1,'ChannelNo',1,'Parameters',struct('DataFileSupport',struct('DataFileSelectedMaster',0,'DataFileSelectedLocal',0,'DataFileName','','DataFileDate','','SelectedFile',['<no file selected>']),'Options',struct('StatusSelected',1,'TimeSelected',1,'DeltaTimeSelected',1,'BytePortSelected',0,'MessageLengthSelected',0,'TriggerPort',struct('Selected',0,'TriggerType','rising'),'UserCoding',struct('Selected',0,'InterfaceFile','UserDecodingFile','FcnName','UserDecodeFcn','InportSelected',0,'InportWidth',1,'OutportSelected',0,'OutportWidth',1),'EnablePortSelected',0,'SignalOnPortnameSelected',1,'UseRXService',0),'Message',struct('MsgOnBlocknameSelected',0,'MsgName',['RX Message'],'MsgIdFormat',0,'MsgId',100,'MsgLength',8,'NumSignals',1,'SampleTime',-1,'Signal',struct('SgnName',['RX signal'],'SgnStartBit',0,'SgnLength',8,'SgnType',0,'ModeValue',-1,'DataType',0,'SLDataType','SS_DOUBLE','ByteLayout',0,'Factor',1,'Offset',0,'Min',0,'Max',255,'SgnComment',{{}},'SgnUnit',''),'MsgIdNumFormat',0,'MsgComment',{{''}}),'Version',1.2,'general',struct('isFromLib',1)),'GroupId',struct('Group',{{'RTICAN'}},'No',1,'Behavior',{{'NAMECHANGE'}},'BlockType',{{'SINK'}},'NameChangeFlag',0),'SFcnRTICANMessage',struct('MsgType','RX','MsgName',['RX Message'],'MsgIdFormat','STD','MsgId',100,'MsgLength',8,'NumSignals',1,'SampleTime',-1,'Signal',struct('SgnName',['RX signal'],'SgnStartBit',0,'SgnLength',8,'SgnType','standard','ModeValue',-1,'DataType',['unsigned int'],'ByteLayout',['little endian'],'SLDataType','SS_DOUBLE','Factor',1,'Offset',0),'StatusSelected','yes','TimeSelected','yes','DeltaTimeSelected','yes','BytePortSelected','no','MessageLengthSelected','no','EnablePortSelected','no','UserCoding',struct('Selected','no','InterfaceFile','UserDecodingFile','FcnName','UserDecodeFcn','InportSelected','no','InportWidth',1,'OutportSelected','no','OutportWidth',1),'TriggerPort',struct('Selected','no','TriggerType','rising'),'UseRXService','no','BoardType','DS4302','BoardNo',1,'ControllerNo',1,'SFcnPortType','Scalar'),'TLCFileName','rtican_rx_message')
      settings: AttributesFormatString=Group Id: RTICAN5\n
  PPEI_VICM_General_Status_11 : rtican/RTICAN Receive (RX)   SystemSampleTime=-1  Reserved1=[]  Reserved2=[]  Reserved3=[]  Reserved4=[]  SfcnMessage=[]  Msg_Struct=[]  BoardTypeNo=[]  BoardNo=[]  ChannelNo=[]  Parameters=[]  DialogFcn=[]  UnitName=[]  Revision=[]  UnitValues=[]  DSProperties=struct('RTI',struct('Version',uint32(5),'BlockType',struct('isSLSource',uint8(1),'isSLSink',uint8(1),'isHWSource',uint8(0),'isHWSink',uint8(0),'isSetup',uint8(0),'isInline',uint8(1),'isNonInline',uint8(0),'isInterrupt',uint8(0),'isChannelwise',uint8(0)),'IOBoardType','RTICAN','UnitType','MESSAGE','Identifier','RX','DialogType','MSVC','BlockSet','RTICAN','SlaveProcessor','CAN'))  RTIBlockInterface=struct('OutputPortsWidth',int32([1 1 1 1 1 1 1 1 1 1 1 1 1 1 1 1 1 1 1 1 1]),'OutputPortsActive',[1 1 1 1 1 1 1 1 1 1 1 1 1 1 1 1 1 1 1 1 1],'OutputPortsName',{{'HVBatPrcdCrnt','HVBatPrcdCrntV','OATEmsnsRelCrVal','ChrgrCntctrStatus','HVChrgrLVPwrSplyStat','HVCntctrStatARC','HVBatFltSevrtyStat','OtsAirTmpEmsnsRel','OtsAirTmpEmsnsRelV','OATEmsnsRelCrValV','OATEmsnsRelCrValM','PrplsnRelBusHVAlwdARC','RefuelVntRqd','PltfrmGenEnStpReq','PrplsnRelBusHVAlwd','FuelDrPosV','FuelDrPos','HVCntctrStat','HVCntctrShdwnReq','ScndHdStatV','ScndHdStat'}},'OutputPortsDataType',{{'SS_DOUBLE','SS_DOUBLE','SS_DOUBLE','SS_DOUBLE','SS_DOUBLE','SS_DOUBLE','SS_DOUBLE','SS_DOUBLE','SS_DOUBLE','SS_DOUBLE','SS_DOUBLE','SS_DOUBLE','SS_DOUBLE','SS_DOUBLE','SS_DOUBLE','SS_DOUBLE','SS_DOUBLE','SS_DOUBLE','SS_DOUBLE','SS_DOUBLE','SS_DOUBLE'}},'OutputPortsLabel',{{'HVBatPrcdCrnt','HVBatPrcdCrntV','OATEmsnsRelCrVal','ChrgrCntctrStatus','HVChrgrLVPwrSplyStat','HVCntctrStatARC','HVBatFltSevrtyStat','OtsAirTmpEmsnsRel','OtsAirTmpEmsnsRelV','OATEmsnsRelCrValV','OATEmsnsRelCrValM','PrplsnRelBusHVAlwdARC','RefuelVntRqd','PltfrmGenEnStpReq','PrplsnRelBusHVAlwd','FuelDrPosV','FuelDrPos','HVCntctrStat','HVCntctrShdwnReq','ScndHdStatV','ScndHdStat'}},'OutputPortsLabelMode','ON','InputPortsWidth',int32(0),'InputPortsActive',0,'DialogFcn','rtican_message_interface_gui','BlockDisplay',{{'','center'}},'IconTransparency','on','ParameterTunableNames',{{}},'InitLevel',3,'BlockName',struct('Token',{{'PPEI_VICM_General_Status_1'}}),'SampleTime',{{-1}},'TriggerPort',{{'none'}},'EnablePort',{{'none'}})  RTIBlockParameters=struct('BoardTypeNo',{{4302,'OFF',[]}},'BoardNo',{{1,'ON',[1 16]}},'ChannelNo',{{2,'ON',[1 4]}},'Parameters',{{struct('DataFileSupport',struct('DataFileSelectedMaster',1,'DataFileSelectedLocal',1,'DataFileName',['c:\data\databases\6.4.1\globala - pe.dbc|'],'DataFileDate',['24-Apr-2014 15:33:48'],'SelectedFile',['..\databases\8.4.5 (140425)\globala - pe.dbc'],'InterfaceFcn','rtican_dbc_file_parser'),'Options',struct('StatusSelected',0,'TimeSelected',0,'DeltaTimeSelected',0,'BytePortSelected',0,'MessageLengthSelected',0,'TriggerPort',struct('Selected',0,'TriggerType',0),'UserCoding',struct('Selected',0,'InterfaceFile','UserDecodingFile','FcnName','UserDecodeFcn','InportSelected',0,'InportWidth',1,'OutportSelected',0,'OutportWidth',1),'EnablePortSelected',0,'SignalOnPortnameSelected',1,'UseRXService',0),'Message',struct('MsgOnBlocknameSelected',1,'MsgName','PPEI_VICM_General_Status_1','MsgIdFormat',0,'MsgId',472,'MsgLength',8,'NumSignals',21,'SampleTime',-1,'Signal',struct('SgnName',{'HVBatPrcdCrnt','HVBatPrcdCrntV','OATEmsnsRelCrVal','ChrgrCntctrStatus','HVChrgrLVPwrSplyStat','HVCntctrStatARC','HVBatFltSevrtyStat','OtsAirTmpEmsnsRel','OtsAirTmpEmsnsRelV','OATEmsnsRelCrValV','OATEmsnsRelCrValM','PrplsnRelBusHVAlwdARC','RefuelVntRqd','PltfrmGenEnStpReq','PrplsnRelBusHVAlwd','FuelDrPosV','FuelDrPos','HVCntctrStat','HVCntctrShdwnReq','ScndHdStatV','ScndHdStat'},'SgnStartBit',{0,12,16,24,27,28,30,32,40,41,42,43,47,48,51,53,54,56,59,61,62},'SgnLength',{12,1,8,3,1,2,2,8,1,1,1,2,1,3,1,1,2,3,2,1,2},'ByteLayout',{2,2,2,2,2,2,2,2,2,2,2,2,2,2,2,2,2,2,2,2,2},'Factor',{0.3,1,0.5,1,1,1,1,0.5,1,1,1,1,1,1,1,1,1,1,1,1,1},'Offset',{0,0,-40,0,0,0,0,-40,0,0,0,0,0,0,0,0,0,0,0,0,0},'SgnComment',{'','','','','','','','','','','','','','','','','','','','',''},'SgnUnit',{'Amps','',['deg C'],'','','','',['deg C'],'','','','','','','','','','','','',''},'Min',{-614.4,0,-40,0,0,0,0,-40,0,0,0,0,0,0,0,0,0,0,0,0,0},'Max',{614.1,1,87.5,7,1,3,3,87.5,1,1,1,3,1,7,1,1,3,7,3,1,3},'SgnType',{0,0,0,0,0,0,0,0,0,0,0,0,0,0,0,0,0,0,0,0,0},'SLDataType',{'SS_DOUBLE','SS_DOUBLE','SS_DOUBLE','SS_DOUBLE','SS_DOUBLE','SS_DOUBLE','SS_DOUBLE','SS_DOUBLE','SS_DOUBLE','SS_DOUBLE','SS_DOUBLE','SS_DOUBLE','SS_DOUBLE','SS_DOUBLE','SS_DOUBLE','SS_DOUBLE','SS_DOUBLE','SS_DOUBLE','SS_DOUBLE','SS_DOUBLE','SS_DOUBLE'},'DataType',{1,0,0,0,0,0,0,0,0,0,0,0,0,0,0,0,0,0,0,0,0},'ModeValue',{-1,-1,-1,-1,-1,-1,-1,-1,-1,-1,-1,-1,-1,-1,-1,-1,-1,-1,-1,-1,-1}),'MsgIdNumFormat',0,'MsgComment',{{''}}),'Version',1.2,'general',struct('isFromLib',0)),'OFF',[]}},'GroupId',{{struct('Group',{{'RTICAN'}},'No',5,'Behavior',{{'NAMECHANGE'}},'BlockType',{{'SINK'}},'NameChangeFlag',0),'OFF',[]}},'SFcnRTICANMessage',{{struct('MsgType','RX','SFcnPortType','Scalar','MsgName','PPEI_VICM_General_Status_1','MsgIdFormat','STD','MsgId',472,'MsgLength',8,'NumSignals',21,'SampleTime',-1,'Signal',struct('SgnName',{'HVBatPrcdCrnt','HVBatPrcdCrntV','OATEmsnsRelCrVal','ChrgrCntctrStatus','HVChrgrLVPwrSplyStat','HVCntctrStatARC','HVBatFltSevrtyStat','OtsAirTmpEmsnsRel','OtsAirTmpEmsnsRelV','OATEmsnsRelCrValV','OATEmsnsRelCrValM','PrplsnRelBusHVAlwdARC','RefuelVntRqd','PltfrmGenEnStpReq','PrplsnRelBusHVAlwd','FuelDrPosV','FuelDrPos','HVCntctrStat','HVCntctrShdwnReq','ScndHdStatV','ScndHdStat'},'SgnStartBit',{0,12,16,24,27,28,30,32,40,41,42,43,47,48,51,53,54,56,59,61,62},'SgnLength',{12,1,8,3,1,2,2,8,1,1,1,2,1,3,1,1,2,3,2,1,2},'ByteLayout',{['motorola back.'],['motorola back.'],['motorola back.'],['motorola back.'],['motorola back.'],['motorola back.'],['motorola back.'],['motorola back.'],['motorola back.'],['motorola back.'],['motorola back.'],['motorola back.'],['motorola back.'],['motorola back.'],['motorola back.'],['motorola back.'],['motorola back.'],['motorola back.'],['motorola back.'],['motorola back.'],['motorola back.']},'Factor',{0.3,1,0.5,1,1,1,1,0.5,1,1,1,1,1,1,1,1,1,1,1,1,1},'Offset',{0,0,-40,0,0,0,0,-40,0,0,0,0,0,0,0,0,0,0,0,0,0},'SgnType',{'standard','standard','standard','standard','standard','standard','standard','standard','standard','standard','standard','standard','standard','standard','standard','standard','standard','standard','standard','standard','standard'},'SLDataType',{'SS_DOUBLE','SS_DOUBLE','SS_DOUBLE','SS_DOUBLE','SS_DOUBLE','SS_DOUBLE','SS_DOUBLE','SS_DOUBLE','SS_DOUBLE','SS_DOUBLE','SS_DOUBLE','SS_DOUBLE','SS_DOUBLE','SS_DOUBLE','SS_DOUBLE','SS_DOUBLE','SS_DOUBLE','SS_DOUBLE','SS_DOUBLE','SS_DOUBLE','SS_DOUBLE'},'DataType',{['signed int'],['unsigned int'],['unsigned int'],['unsigned int'],['unsigned int'],['unsigned int'],['unsigned int'],['unsigned int'],['unsigned int'],['unsigned int'],['unsigned int'],['unsigned int'],['unsigned int'],['unsigned int'],['unsigned int'],['unsigned int'],['unsigned int'],['unsigned int'],['unsigned int'],['unsigned int'],['unsigned int']},'ModeValue',{-1,-1,-1,-1,-1,-1,-1,-1,-1,-1,-1,-1,-1,-1,-1,-1,-1,-1,-1,-1,-1}),'StatusSelected','no','TimeSelected','no','DeltaTimeSelected','no','BytePortSelected','no','MessageLengthSelected','no','TriggerPort',struct('Selected','no','TriggerType',0),'UserCoding',struct('Selected','no','InterfaceFile','UserDecodingFile','FcnName','UserDecodeFcn','InportSelected','no','InportWidth',1,'OutportSelected','no','OutportWidth',1),'EnablePortSelected','no','UseRXService','no','BoardType','DS4302','BoardNo',1,'ControllerNo',2),'OFF',[]}},'TLCFileName',{{'rtican_rx_message','OFF',[]}})  RTISFcnParameters=struct('SFcnRTICANMessage','struct','TLCFileName','char')  RTIBlockParaDefault=struct('BoardTypeNo',4302,'BoardNo',1,'ChannelNo',1,'Parameters',struct('DataFileSupport',struct('DataFileSelectedMaster',0,'DataFileSelectedLocal',0,'DataFileName','','DataFileDate','','SelectedFile',['<no file selected>']),'Options',struct('StatusSelected',1,'TimeSelected',1,'DeltaTimeSelected',1,'BytePortSelected',0,'MessageLengthSelected',0,'TriggerPort',struct('Selected',0,'TriggerType','rising'),'UserCoding',struct('Selected',0,'InterfaceFile','UserDecodingFile','FcnName','UserDecodeFcn','InportSelected',0,'InportWidth',1,'OutportSelected',0,'OutportWidth',1),'EnablePortSelected',0,'SignalOnPortnameSelected',1,'UseRXService',0),'Message',struct('MsgOnBlocknameSelected',0,'MsgName',['RX Message'],'MsgIdFormat',0,'MsgId',100,'MsgLength',8,'NumSignals',1,'SampleTime',-1,'Signal',struct('SgnName',['RX signal'],'SgnStartBit',0,'SgnLength',8,'SgnType',0,'ModeValue',-1,'DataType',0,'SLDataType','SS_DOUBLE','ByteLayout',0,'Factor',1,'Offset',0,'Min',0,'Max',255,'SgnComment',{{}},'SgnUnit',''),'MsgIdNumFormat',0,'MsgComment',{{''}}),'Version',1.2,'general',struct('isFromLib',1)),'GroupId',struct('Group',{{'RTICAN'}},'No',1,'Behavior',{{'NAMECHANGE'}},'BlockType',{{'SINK'}},'NameChangeFlag',0),'SFcnRTICANMessage',struct('MsgType','RX','MsgName',['RX Message'],'MsgIdFormat','STD','MsgId',100,'MsgLength',8,'NumSignals',1,'SampleTime',-1,'Signal',struct('SgnName',['RX signal'],'SgnStartBit',0,'SgnLength',8,'SgnType','standard','ModeValue',-1,'DataType',['unsigned int'],'ByteLayout',['little endian'],'SLDataType','SS_DOUBLE','Factor',1,'Offset',0),'StatusSelected','yes','TimeSelected','yes','DeltaTimeSelected','yes','BytePortSelected','no','MessageLengthSelected','no','EnablePortSelected','no','UserCoding',struct('Selected','no','InterfaceFile','UserDecodingFile','FcnName','UserDecodeFcn','InportSelected','no','InportWidth',1,'OutportSelected','no','OutportWidth',1),'TriggerPort',struct('Selected','no','TriggerType','rising'),'UseRXService','no','BoardType','DS4302','BoardNo',1,'ControllerNo',1,'SFcnPortType','Scalar'),'TLCFileName','rtican_rx_message')
      settings: AttributesFormatString=Group Id: RTICAN5\n
  Terminator{,1..4,6..12} (12 alike) : Terminator
  Terminator_{1..5,13..31,33,35..36} (27 alike) : Terminator
  LT_PwrDschLmt : Outport  OutDataType=sfix(16)  OutScaling=2^0
  LT_PwrChgLmt : Outport  Port=2  OutDataType=sfix(16)  OutScaling=2^0
  SOC : Outport  Port=3  OutDataType=sfix(16)  OutScaling=2^0
  Voltage : Outport  Port=4  OutDataType=sfix(16)  OutScaling=2^0
  PackCurrent : Outport  Port=5  OutDataType=sfix(16)  OutScaling=2^0
  ContactorStatus : Outport  Port=6  OutDataType=sfix(16)  OutScaling=2^0
  HVBatVltUpLmt_CAN : Outport  Port=7  OutDataType=sfix(16)  OutScaling=2^0
  HVBatVltLwLmt_CAN : Outport  Port=8  OutDataType=sfix(16)  OutScaling=2^0
  HVBatCrntLwLmt_CAN : Outport  Port=9  OutDataType=sfix(16)  OutScaling=2^0
  HVBatCrntUpLmt_CAN : Outport  Port=10  OutDataType=sfix(16)  OutScaling=2^0
  wires:
  PPEI_High_Volt_Batt_Dchrg_Pwrs1/1 -> Terminator/1  "HVBDP_ShrtTrmDischrgPwr"
  PPEI_High_Volt_Batt_Dchrg_Pwrs1/2 -> Terminator2/1  "HVBDP_CrnkDischrgPwrV"
  PPEI_High_Volt_Batt_Dchrg_Pwrs1/3 -> Terminator3/1  "HVBDP_Res"
  PPEI_High_Volt_Batt_Dchrg_Pwrs1/4 -> LT_PwrDschLmt/1  "HVBDP_LngTrmDischrgPwr"
  PPEI_High_Volt_Batt_Dchrg_Pwrs1/5 -> Terminator6/1  "HVBDP_CrnkDischrgPwr"
  PPEI_High_Voltage_Batt_Chrg_Pwrs1/1 -> SOC/1  "HVBatSOCHiRes"
  PPEI_High_Voltage_Batt_Chrg_Pwrs1/2 -> Terminator7/1  "HVBatOutOfEnrgyStat"
  PPEI_High_Voltage_Batt_Chrg_Pwrs1/3 -> Terminator8/1  "HVBatSOCHiResV"
  PPEI_High_Voltage_Batt_Chrg_Pwrs1/4 -> Terminator9/1  "HVBCP_ShrtTrmChrgPwr"
  PPEI_High_Voltage_Batt_Chrg_Pwrs1/5 -> Terminator10/1  "HVBCP_CrnkChrgPwrV"
  PPEI_High_Voltage_Batt_Chrg_Pwrs1/6 -> Terminator11/1  "HVBCP_Res"
  PPEI_High_Voltage_Batt_Chrg_Pwrs1/8 -> Terminator12/1  "HVBCP_CrnkChrgPwr"
  PPEI_High_Voltage_Batt_Chrg_Pwrs1/7 -> LT_PwrChgLmt/1  "HVBCP_LngTrmChrgPwr"
  PPEI_VICM_General_Status_11/1 -> PackCurrent/1  "HVBatPrcdCrnt"
  PPEI_VICM_General_Status_11/18 -> ContactorStatus/1  "HVCntctrStat"
  PPEI_VICM_General_Status_11/2 -> Terminator_13/1  "HVBatPrcdCrntV"
  PPEI_VICM_General_Status_11/3 -> Terminator_14/1  "OATEmsnsRelCrVal"
  PPEI_VICM_General_Status_11/4 -> Terminator_15/1  "ChrgrCntctrStatus"
  PPEI_VICM_General_Status_11/5 -> Terminator_16/1  "HVChrgrLVPwrSplyStat"
  PPEI_VICM_General_Status_11/6 -> Terminator_17/1  "HVCntctrStatARC"
  PPEI_VICM_General_Status_11/8 -> Terminator_18/1  "OtsAirTmpEmsnsRel"
  PPEI_VICM_General_Status_11/9 -> Terminator_19/1  "OtsAirTmpEmsnsRelV"
  PPEI_VICM_General_Status_11/10 -> Terminator_20/1  "OATEmsnsRelCrValV"
  PPEI_VICM_General_Status_11/11 -> Terminator_21/1  "OATEmsnsRelCrValM"
  PPEI_VICM_General_Status_11/13 -> Terminator_22/1  "RefuelVntRqd"
  PPEI_VICM_General_Status_11/16 -> Terminator_25/1  "FuelDrPosV"
  PPEI_VICM_General_Status_11/17 -> Terminator_26/1  "FuelDrPos"
  PPEI_VICM_General_Status_11/19 -> Terminator_27/1  "HVCntctrShdwnReq"
  PPEI_VICM_General_Status_11/20 -> Terminator_28/1  "ScndHdStatV"
  PPEI_VICM_General_Status_11/21 -> Terminator_29/1  "ScndHdStat"
  PPEI_High_Vlt_Battery_Vlt_Status1/7 -> Voltage/1  "HVBatPackPrcdVltg"
  PPEI_High_Vlt_Battery_Vlt_Status1/1 -> Terminator_30/1  "HVBatVltLwLmtCrnk"
  PPEI_High_Vlt_Battery_Vlt_Status1/2 -> Terminator_31/1  "HVBatVltLwLmtCrnkV"
  PPEI_High_Vlt_Battery_Vlt_Status1/3 -> HVBatVltLwLmt_CAN/1  "HVBatVltLwLmt"
  PPEI_High_Vlt_Battery_Vlt_Status1/4 -> Terminator_33/1  "HVBatVltLwLmtV"
  PPEI_High_Vlt_Battery_Vlt_Status1/5 -> HVBatVltUpLmt_CAN/1  "HVBatVltUpLmt"
  PPEI_High_Vlt_Battery_Vlt_Status1/6 -> Terminator_35/1  "HVBatVltUpLmtV"
  PPEI_High_Vlt_Battery_Vlt_Status1/8 -> Terminator_36/1  "HVBatPackPrcdVltgV"
  PPEI_High_Volt_Batt_Current_Stat1/1 -> Terminator_1/1  "HVBatStOfChrgMin"
  PPEI_High_Volt_Batt_Current_Stat1/2 -> HVBatCrntLwLmt_CAN/1  "HVBatCrntLwLmt"
  PPEI_High_Volt_Batt_Current_Stat1/3 -> Terminator_3/1  "HVBatCrntLwLmtV"
  PPEI_High_Volt_Batt_Current_Stat1/4 -> HVBatCrntUpLmt_CAN/1  "HVBatCrntUpLmt"
  PPEI_High_Volt_Batt_Current_Stat1/5 -> Terminator_4/1  "HVBatCrntUpLmtV"
